simulink model "stm32"  (R2024b)
settings: Solver=FixedStepAuto  StartTime=0.0  StopTime=10.0  RelTol=1e-3  EnableMultiTasking=on
libraries: stm32f4xxblockslib x15
settings Model: STM32="{\"AnalogInput\":[{\"ID\":\"untitled:32\"},{\"ID\":\"untitled:47\"},{\"ID\":\"untitled:48\"}],\"DigitalPortRead\":[{\"ID\":\"untitled:35\"},{\"ID\":\"untitled:36\"},{\"ID\":\"untitled:37\"},{\"ID\":\"stm32:75\"},{\"ID\":\"stm32:76\"},{\"ID\":\"stm32:77\"},{\"ID\":\"stm32:86\"},{\"ID\":\"stm32:87\"},{\"ID\":\"stm32:88\"}],\"DigitalPortWrite\":[{\"ID\":\"untitled:38\"},{\"ID\":\"untitled:39\"},{\"ID\":\"untitled:40\"},{\"ID\":\"untitled:41\"},{\"ID\":\"untitled:42\"},{\"ID\":\"untitled:43\"},{\"ID\":\"untitled:44\"},{\"ID\":\"untitled:45\"},{\"ID\":\"untitled:46\"},{\"ID\":\"stm32:63\"},{\"ID\":\"stm32:64\"},{\"ID\":\"stm32:65\"},{\"ID\":\"stm32:66\"},{\"ID\":\"stm32:67\"},{\"ID\":\"stm32:68\"},{\"ID\":\"stm32:69\"},{\"ID\":\"stm32:70\"},{\"ID\":\"stm32:71\"}]}"  SimulationMode=external  Creator=chall  LastModifiedBy=chall
settings OptimizationCC: DefaultParameterBehavior=Inlined  EnhancedBackFolding=on  PassReuseOutputArgsAs=Individual arguments  ZeroExternalMemoryAtStartup=off  ZeroInternalMemoryAtStartup=off  MaxStackSize=512  OptimizeBlockOrder=speed  DifferentSizesBufferReuse=on  OptimizationCustomize=off  EfficientTunableParamExpr=on
settings DebuggingCC: ParameterTunabilityLossMsg=error
settings HardwareCC: ProdBitPerPointer=32  ProdBitPerSizeT=32  ProdBitPerPtrDiffT=32  ProdLargestAtomicInteger=Long  ProdLargestAtomicFloat=Double  ProdWordSize=32  ProdLongLongMode=on  ProdHWDeviceType=ARM Compatible->ARM Cortex-M
settings SFSimCC: MATLABDynamicMemAlloc=off
settings RTWCC: Description=Embedded Coder  SystemTargetFile=ert.tlc  HardwareBoard=STM32F4xx Based  TemplateMakefile=ert_default_tmf  Toolchain=GNU Tools for ARM Embedded Processors
settings CodeAppCC: ForceParamTrailComments=on  IgnoreCustomStorageClasses=off  OperatorAnnotations=on  SimulinkDataObjDesc=on  SFDataObjDesc=on  InsertBlockDesc=on
settings ERTTargetCC: TargetLangStandard=C99 (ISO)  CodeReplacementLibrary=ARM Cortex-M  ExtModeTransport=3  ExtModeStaticAlloc=on  ExtModeStaticAllocSize=2048  ExtModeMexFile=ext_xcp  ExtModeIntrfLevel=Level2 - Open

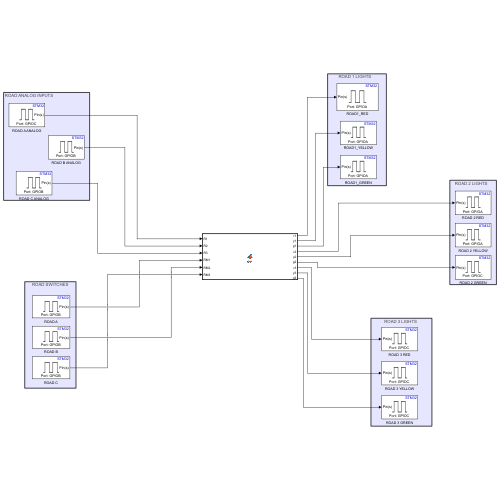
[thumbnail: Simulink's stored preview of the top-level diagram]
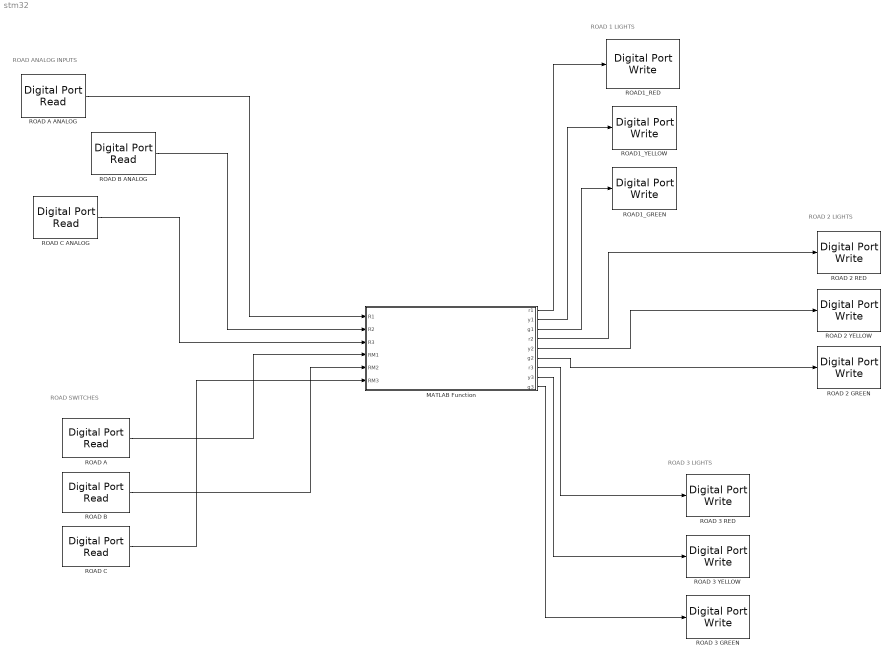
== system stm32 ==
  note: ROAD ANALOG INPUTS
  note: ROAD SWITCHES
  note: ROAD 3 LIGHTS
  note: ROAD 2 LIGHTS
  note: ROAD 1 LIGHTS
  MATLAB Function : MATLAB Function  TreatAsAtomicUnit=on
  ROAD 2 GREEN : stm32f4xxblockslib/Digital Port Write  PortName=GPIOC  PinNumber=9  ReadOperation=off  IOAsArray=on  EnableSimPort=off  hoistedMaskSrc=ECSoC/ECSimCodegen/Digital Port Write
  ROAD 2 RED : stm32f4xxblockslib/Digital Port Write  PortName=GPIOA  PinNumber=9  ReadOperation=off  IOAsArray=on  EnableSimPort=off  hoistedMaskSrc=ECSoC/ECSimCodegen/Digital Port Write
  ROAD 2 YELLOW : stm32f4xxblockslib/Digital Port Write  PortName=GPIOA  PinNumber=8  ReadOperation=off  IOAsArray=on  EnableSimPort=off  hoistedMaskSrc=ECSoC/ECSimCodegen/Digital Port Write
  ROAD 3 GREEN : stm32f4xxblockslib/Digital Port Write  PortName=GPIOC  PinNumber=6  ReadOperation=off  IOAsArray=on  EnableSimPort=off  hoistedMaskSrc=ECSoC/ECSimCodegen/Digital Port Write
  ROAD 3 RED : stm32f4xxblockslib/Digital Port Write  PortName=GPIOC  PinNumber=8  ReadOperation=off  IOAsArray=on  EnableSimPort=off  hoistedMaskSrc=ECSoC/ECSimCodegen/Digital Port Write
  ROAD 3 YELLOW : stm32f4xxblockslib/Digital Port Write  PortName=GPIOC  PinNumber=7  ReadOperation=off  IOAsArray=on  EnableSimPort=off  hoistedMaskSrc=ECSoC/ECSimCodegen/Digital Port Write
  ROAD A : stm32f4xxblockslib/Digital Port Read  PortName=GPIOB  PinNumber=14  ReadOperation=on  IOAsArray=on  SampleTime=-1  EnableSimPort=off  hoistedMaskSrc=ECSoC/ECSimCodegen/Digital Port Read
      settings: LibrarySourceBlock=stm32l4xxblockslib/Digital Port Read
  ROAD A ANALOG : stm32f4xxblockslib/Digital Port Read  PortName=GPIOC  PinNumber=5  ReadOperation=on  IOAsArray=on  SampleTime=-1  EnableSimPort=off  hoistedMaskSrc=ECSoC/ECSimCodegen/Digital Port Read
  ROAD B : stm32f4xxblockslib/Digital Port Read  PortName=GPIOB  PinNumber=13  ReadOperation=on  IOAsArray=on  SampleTime=-1  EnableSimPort=off  hoistedMaskSrc=ECSoC/ECSimCodegen/Digital Port Read
      settings: LibrarySourceBlock=stm32l4xxblockslib/Digital Port Read
  ROAD B ANALOG : stm32f4xxblockslib/Digital Port Read  PortName=GPIOB  PinNumber=0  ReadOperation=on  IOAsArray=on  SampleTime=-1  EnableSimPort=off  hoistedMaskSrc=ECSoC/ECSimCodegen/Digital Port Read
  ROAD C : stm32f4xxblockslib/Digital Port Read  PortName=GPIOB  PinNumber=12  ReadOperation=on  IOAsArray=on  SampleTime=-1  EnableSimPort=off  hoistedMaskSrc=ECSoC/ECSimCodegen/Digital Port Read
      settings: LibrarySourceBlock=stm32l4xxblockslib/Digital Port Read
  ROAD C ANALOG : stm32f4xxblockslib/Digital Port Read  PortName=GPIOB  PinNumber=1  ReadOperation=on  IOAsArray=on  SampleTime=-1  EnableSimPort=off  hoistedMaskSrc=ECSoC/ECSimCodegen/Digital Port Read
  ROAD1_GREEN : stm32f4xxblockslib/Digital Port Write  PortName=GPIOA  PinNumber=10  ReadOperation=off  IOAsArray=on  EnableSimPort=off  hoistedMaskSrc=ECSoC/ECSimCodegen/Digital Port Write
  ROAD1_RED : stm32f4xxblockslib/Digital Port Write  PortName=GPIOA  PinNumber=12  ReadOperation=off  IOAsArray=on  EnableSimPort=off  hoistedMaskSrc=ECSoC/ECSimCodegen/Digital Port Write
  ROAD1_YELLOW : stm32f4xxblockslib/Digital Port Write  PortName=GPIOA  PinNumber=11  ReadOperation=off  IOAsArray=on  EnableSimPort=off  hoistedMaskSrc=ECSoC/ECSimCodegen/Digital Port Write
  wires:
  ROAD A/1 -> MATLAB Function/4(RM1)
  MATLAB Function/3(g1) -> ROAD1_GREEN/1
  MATLAB Function/4(r2) -> ROAD 2 RED/1
  MATLAB Function/5(y2) -> ROAD 2 YELLOW/1
  ROAD C ANALOG/1 -> MATLAB Function/3(R3)
  MATLAB Function/1(r1) -> ROAD1_RED/1
  ROAD B ANALOG/1 -> MATLAB Function/2(R2)
  MATLAB Function/2(y1) -> ROAD1_YELLOW/1
  ROAD A ANALOG/1 -> MATLAB Function/1(R1)
  ROAD C/1 -> MATLAB Function/6(RM3)
  ROAD B/1 -> MATLAB Function/5(RM2)
  MATLAB Function/7(r3) -> ROAD 3 RED/1
  MATLAB Function/9(g3) -> ROAD 3 GREEN/1
  MATLAB Function/8(y3) -> ROAD 3 YELLOW/1
  MATLAB Function/6(g2) -> ROAD 2 GREEN/1

== matlab function stm32/MATLAB Function ==
  data: R1 input; r1 output; R2 input; R3 input; RM1 input; RM2 input; RM3 input; y1 output; g1 output; r2 output; y2 output; g2 output; r3 output; y3 output; g3 output
function [r1,y1,g1,r2,y2,g2,r3,y3,g3] = fcn(R1,R2,R3,RM1,RM2,RM3)


r1 = 0; y1 = 0; g1 = 0;
r2 = 0; y2 = 0; g2 = 0;
r3 = 0; y3 = 0; g3 = 0;


   if R1 > R2 && R1 > R3
        r1 = 0; y1 = 0; g1 = 1;
        r2 = 1; y2 = 0; g2 = 0;
        r3 = 0; y3 = 1; g3 = 0;
    elseif R2 > R3 && R2>R1
        r1 = 0; y1 = 1; g1 = 0;
        r2 = 0; y2 = 0; g2 = 1;
        r3 = 1; y3 = 0; g3 = 0;
    elseif R3 > R1 && R3 > R2
        r1 = 1; y1 = 0; g1 = 0;
        r2 = 0; y2 = 1; g2 = 0;
        r3 = 0; y3 = 0; g3 = 1;
   end

    if RM1 == 1
        r1 = 0; y1 = 0; g1 = 1;
        r2 = 1; y2 = 0; g2 = 0;
        r3 = 0; y3 = 1; g3 = 0;
    elseif RM2 == 1  
        r1 = 0; y1 = 1; g1 = 0;
        r2 = 0; y2 = 0; g2 = 1;
        r3 = 1; y3 = 0; g3 = 0;
    elseif RM3 == 1
        r1 = 1; y1 = 0; g1 = 0;
        r2 = 0; y2 = 1; g2 = 0;
        r3 = 0; y3 = 0; g3 = 1;
   
   
end



end
